simulink model "untitled1"  (R2024b)
settings: Solver=VariableStepAuto  StartTime=0.0  StopTime=10.0  RelTol=1e-3
libraries: shared6dof x1
settings Model: Creator=the_main_notebook  LastModifiedBy=the_main_notebook

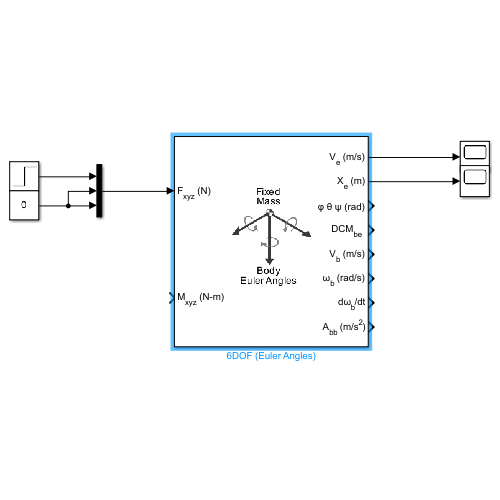
[thumbnail: Simulink's stored preview of the top-level diagram]
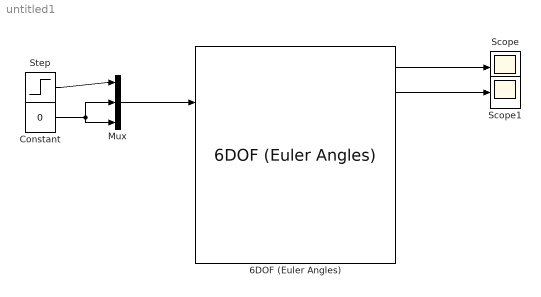
== system untitled1 ==
  6DOF (Euler Angles) : shared6dof/6DOF (Euler Angles)  units=Metric (MKS)  mtype=Fixed  rep=Euler Angles  xme_0=[0 0 0]  Vm_0=[0 0 0]  eul_0=[0 0 0]  pm_0=[0 0 0]  mass_0=1.0  mass_e=0.5  mass_f=2.0  inertia=eye(3)  inertia_e=eye(3)  inertia_f=2*eye(3)  k_quat=1.0  vre_flag=on  abi_flag=off  aMode=0  xme_statename=''  Vm_statename=''  eul_statename=''  quat_statename=''  pm_statename=''  mass_statename=''
  Constant : Constant  Value=0
  Mux : Mux  Inputs=3
  Scope : Scope
  Scope1 : Scope
  Step : Step  After=100  SampleTime=0
  wires:
  6DOF (Euler Angles)/1 -> Scope/1
  Mux/1 -> 6DOF (Euler Angles)/1
  Step/1 -> Mux/1
  Constant/1 -> Mux/2, Mux/3
  6DOF (Euler Angles)/2 -> Scope1/1
